simulink model "MatlabFunction"  (R2015b)
settings: Solver=FixedStepAuto  StartTime=0.0  StopTime=10.0  FixedStep=1  RelTol=1e-3
settings Model: Creator=LUBO  LastModifiedBy=LUBO

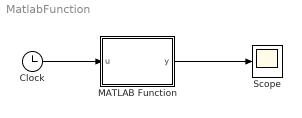
== system MatlabFunction ==
  Clock : Clock
  MATLAB Function : MATLAB Function  TreatAsAtomicUnit=on
  Scope : Scope
  wires:
  Clock/1 -> MATLAB Function/1(u)
  MATLAB Function/1(y) -> Scope/1

== matlab function MatlabFunction/MATLAB Function ==
  data: u input; y output
function y = fcn(u)
%#codegen
persistent sum_val
if isempty(sum_val)
    sum_val=0;
end
sum_val=sum_val+u;
y = sum_val;
